simulink model "compare"  (Simulink 6.6)
settings: Solver=VariableStepDiscrete  StartTime=0.0  StopTime=5  RelTol=1e-3
PreLoadFcn:
  | RRCFilterWeights = [
  |    0.001370231076202
  |    0.002539899911233
  |   -0.003621094462482
  |   -0.000728764715513
  |    0.004498121197526
  |   -0.003650933561409
  |   -0.001434685694509
  |    0.010428163868336
  |   -0.009027836713693
  |   -0.018575100972486
  |    0.032428528983592
  |    0.026411593954204
  |   -0.084942459066375
  |   -0.032083970770240
  |    0.310814941216985
  |    0.534154943091895
  |    0.310814941216985
  |   -0.032083970770240
  |   -0.084942459066375
  |    0.026411593954204
  |    0.032428528983592
  |   -0.018575100972486
  |   -0.009027836713693
  |    0.010428163868336
  |   -0.001434685694509
  |   -0.003650933561409
  |    0.004498121197526
  |   -0.000728764715513
  |   -0.003621094462482
  |    0.002539899911233
  |    0.001370231076202];
StopFcn:
  | doFFTplot((2400*4),[fir],['Upsample-Filter'],1,1,'hann')
  | grid on;
  | 
  | doFFTplot((2400*4),[polyphase],['Polyphase'],1,2,'hann')
  | grid on;
  | 
  | figure(3)
  | subplot(2,1,1)
  | plot(fir(1:100),'k-o','MarkerFaceColor','r');
  | legend('Shaped Pulses (Upsample-Filter)',1');
  | axis([0 100 -1 1]);
  | subplot(2,1,2)
  | plot(polyphase(1:100),'k-o','MarkerFaceColor','b');
  | legend('Shaped Pulses (Polyphase)',1');
  | axis([0 100 -1 1]);
libraries: xbsIndex_r4 x249
(part 3 of 3)

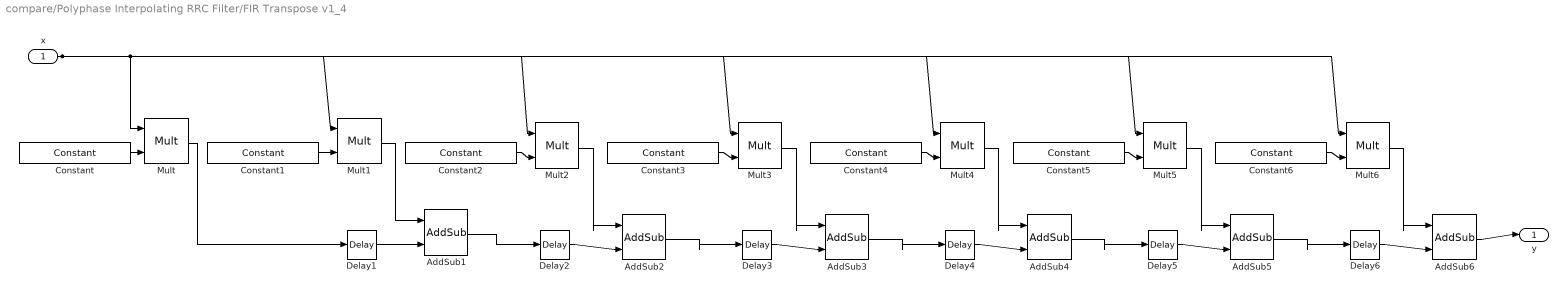
== system compare/Polyphase Interpolating RRC Filter/FIR Transpose v1_4 ==
  x : Inport
  AddSub1 : xbsIndex_r4/AddSub  mode=Addition  use_carryin=off  use_carryout=off  en=off  latency=0  precision=User Defined  arith_type="Signed  (2's comp)"  n_bits=input_bits + coeff_n_bits + 1 + (floor(log2(1)))  bin_pt=input_f_bits+coeff_f_bits  quantization=Truncate  overflow=Wrap  dbl_ovrd=off  use_behavioral_HDL=off  pipelined=off  use_rpm=on  block_type=addsub
      settings: block_version=8.2.01
  AddSub2 : xbsIndex_r4/AddSub  mode=Addition  use_carryin=off  use_carryout=off  en=off  latency=0  precision=User Defined  arith_type="Signed  (2's comp)"  n_bits=input_bits + coeff_n_bits + 1 + (floor(log2(2)))  bin_pt=input_f_bits+coeff_f_bits  quantization=Truncate  overflow=Wrap  dbl_ovrd=off  use_behavioral_HDL=off  pipelined=off  use_rpm=on  block_type=addsub
      settings: block_version=8.2.01
  AddSub3 : xbsIndex_r4/AddSub  mode=Addition  use_carryin=off  use_carryout=off  en=off  latency=0  precision=User Defined  arith_type="Signed  (2's comp)"  n_bits=input_bits + coeff_n_bits + 1 + (floor(log2(3)))  bin_pt=input_f_bits+coeff_f_bits  quantization=Truncate  overflow=Wrap  dbl_ovrd=off  use_behavioral_HDL=off  pipelined=off  use_rpm=on  block_type=addsub
      settings: block_version=8.2.01
  AddSub4 : xbsIndex_r4/AddSub  mode=Addition  use_carryin=off  use_carryout=off  en=off  latency=0  precision=User Defined  arith_type="Signed  (2's comp)"  n_bits=input_bits + coeff_n_bits + 1 + (floor(log2(4)))  bin_pt=input_f_bits+coeff_f_bits  quantization=Truncate  overflow=Wrap  dbl_ovrd=off  use_behavioral_HDL=off  pipelined=off  use_rpm=on  block_type=addsub
      settings: block_version=8.2.01
  AddSub5 : xbsIndex_r4/AddSub  mode=Addition  use_carryin=off  use_carryout=off  en=off  latency=0  precision=User Defined  arith_type="Signed  (2's comp)"  n_bits=input_bits + coeff_n_bits + 1 + (floor(log2(5)))  bin_pt=input_f_bits+coeff_f_bits  quantization=Truncate  overflow=Wrap  dbl_ovrd=off  use_behavioral_HDL=off  pipelined=off  use_rpm=on  block_type=addsub
      settings: block_version=8.2.01
  AddSub6 : xbsIndex_r4/AddSub  mode=Addition  use_carryin=off  use_carryout=off  en=off  latency=0  precision=User Defined  arith_type="Signed  (2's comp)"  n_bits=input_bits + coeff_n_bits + 1 + (floor(log2(6)))  bin_pt=input_f_bits+coeff_f_bits  quantization=Truncate  overflow=Wrap  dbl_ovrd=off  use_behavioral_HDL=off  pipelined=off  use_rpm=on  block_type=addsub
      settings: block_version=8.2.01
  Constant : xbsIndex_r4/Constant  arith_type=Signed (2's comp)  const=coef(7)  n_bits=coeff_n_bits  bin_pt=coeff_f_bits  explicit_period=off  period=1  equ=P=C  opselect=C  inp2=PCIN>>17  opr=+  inp1=P  carry=CIN  dbl_ovrd=off  block_type=constant
      settings: block_version=8.2.01
  Constant1 : xbsIndex_r4/Constant  arith_type=Signed (2's comp)  const=coef(6)  n_bits=coeff_n_bits  bin_pt=coeff_f_bits  explicit_period=off  period=1  equ=P=C  opselect=C  inp2=PCIN>>17  opr=+  inp1=P  carry=CIN  dbl_ovrd=off  block_type=constant
      settings: block_version=8.2.01
  Constant2 : xbsIndex_r4/Constant  arith_type=Signed (2's comp)  const=coef(5)  n_bits=coeff_n_bits  bin_pt=coeff_f_bits  explicit_period=off  period=1  equ=P=C  opselect=C  inp2=PCIN>>17  opr=+  inp1=P  carry=CIN  dbl_ovrd=off  block_type=constant
      settings: block_version=8.2.01
  Constant3 : xbsIndex_r4/Constant  arith_type=Signed (2's comp)  const=coef(4)  n_bits=coeff_n_bits  bin_pt=coeff_f_bits  explicit_period=off  period=1  equ=P=C  opselect=C  inp2=PCIN>>17  opr=+  inp1=P  carry=CIN  dbl_ovrd=off  block_type=constant
      settings: block_version=8.2.01
  Constant4 : xbsIndex_r4/Constant  arith_type=Signed (2's comp)  const=coef(3)  n_bits=coeff_n_bits  bin_pt=coeff_f_bits  explicit_period=off  period=1  equ=P=C  opselect=C  inp2=PCIN>>17  opr=+  inp1=P  carry=CIN  dbl_ovrd=off  block_type=constant
      settings: block_version=8.2.01
  Constant5 : xbsIndex_r4/Constant  arith_type=Signed (2's comp)  const=coef(2)  n_bits=coeff_n_bits  bin_pt=coeff_f_bits  explicit_period=off  period=1  equ=P=C  opselect=C  inp2=PCIN>>17  opr=+  inp1=P  carry=CIN  dbl_ovrd=off  block_type=constant
      settings: block_version=8.2.01
  Constant6 : xbsIndex_r4/Constant  arith_type=Signed (2's comp)  const=coef(1)  n_bits=coeff_n_bits  bin_pt=coeff_f_bits  explicit_period=off  period=1  equ=P=C  opselect=C  inp2=PCIN>>17  opr=+  inp1=P  carry=CIN  dbl_ovrd=off  block_type=constant
      settings: block_version=8.2.01
  Delay{1..6} (6 alike) : xbsIndex_r4/Delay  en=off  latency=1  dbl_ovrd=off  reg_retiming=off  block_type=delay
      settings: infoedit=Hardware notes: A delay line is a chain, each link of which is an SRL16 followed by a flip-flop. If register retiming is enabled, the delay line is a chain of flip-flops.  block_version=8.2.01
  Mult{,1..6} (7 alike) : xbsIndex_r4/Mult  precision=User Defined  arith_type="Signed  (2's comp)"  n_bits=input_bits+coeff_n_bits  bin_pt=input_f_bits+coeff_f_bits  quantization=Truncate  overflow=Wrap  en=off  latency=0  dbl_ovrd=off  use_behavioral_HDL=off  use_embedded=on  opt=Speed  optimum_pipeline=off  pipeline=on  use_rpm=on  placement_style=Rectangular shape  block_type=mult
      settings: infoedit=Hardware notes: To use the internal pipeline stage of the dedicated multiplier you must select 'Pipeline for maximum performance'.  block_version=8.2.01
  y : Outport
  wires:
  Delay1/1 -> AddSub1/2
  Mult1/1 -> AddSub1/1
  Mult/1 -> Delay1/1
  Constant1/1 -> Mult1/2
  Constant/1 -> Mult/2
  x/1 -> Mult1/1, Mult/1, Mult2/1, Mult3/1, Mult4/1, Mult5/1, Mult6/1
  Constant2/1 -> Mult2/2
  AddSub1/1 -> Delay2/1
  Delay2/1 -> AddSub2/2
  Mult2/1 -> AddSub2/1
  Constant3/1 -> Mult3/2
  AddSub2/1 -> Delay3/1
  Delay3/1 -> AddSub3/2
  Mult3/1 -> AddSub3/1
  Constant4/1 -> Mult4/2
  AddSub3/1 -> Delay4/1
  Delay4/1 -> AddSub4/2
  Mult4/1 -> AddSub4/1
  Constant5/1 -> Mult5/2
  AddSub4/1 -> Delay5/1
  Delay5/1 -> AddSub5/2
  Mult5/1 -> AddSub5/1
  Constant6/1 -> Mult6/2
  AddSub5/1 -> Delay6/1
  Delay6/1 -> AddSub6/2
  Mult6/1 -> AddSub6/1
  AddSub6/1 -> y/1
